simulink model "joystick_and_autonomous_control"  (Simulink 8.2)
settings: Solver=FixedStepDiscrete  StartTime=0.0  StopTime=inf  FixedStep=0.04  RelTol=1e-3
libraries: etargetslib x17, simulink x13, dspnetwork x11, dspmtrx3 x10, xpcseriallib x7, visionsinks x2, visionstatistics x1, visiontextngfix x1, aerolibanimutils x1, SimulinkExecutionControl x1, instrumentlib x1
(part 1 of 2)
settings Model: Creator=Ballistyx  LastModifiedBy=menkh
settings DebuggingCC: MultiTaskDSMMsg=warning  MultiTaskCondExecSysMsg=none  FcnCallInpInsideContextMsg=EnableAllAsWarning
settings RTWCC: IncludeERTFirstTime=on
settings GRTTargetCC: CombineOutputUpdateFcns=on  GRTInterface=off

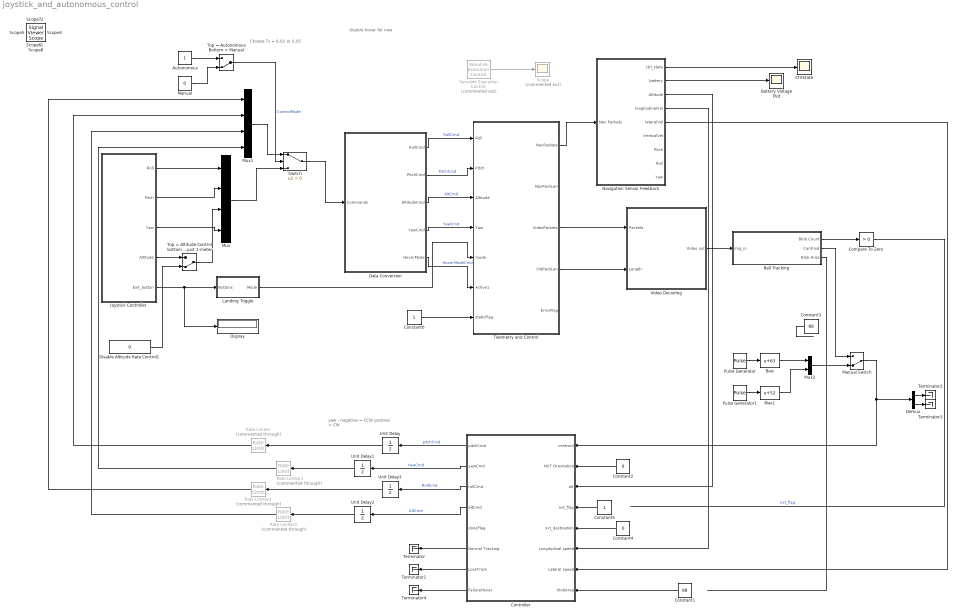
== system joystick_and_autonomous_control ==
  note: Choose Ts = 0.02 or 0.05
  note: yaw - negative = CCW
      | positive = CW
  note: disable hover for now
  Autonomous : Constant
  Ball Tracking : Subsystem
  Battery Voltage Plot : Scope
  Bias : Bias  Bias=63
  Bias1 : Bias  Bias=52  SaturateOnIntegerOverflow=on
  Compare To Zero : simulink/Logic and Bit Operations/Compare To Zero  relop=>  OutDataTypeStr=boolean
  Constant1 : Constant  Value=88
  Constant2 : Constant  Value=0
  Constant3 : Constant  Value=88
  Constant4 : Constant  Value=0  OutDataTypeStr=boolean
  Constant5 : Constant  OutDataTypeStr=boolean
  Constant6 : Constant  OutDataTypeStr=boolean
  "Controller " : Subsystem
  CtrlState : Scope
      settings: YMin=124518  YMax=137626  SaveName=ScopeData2
  Data Conversion : Subsystem
  Demux : Demux  Outputs=2
  Disable Altitude Rate Control1 : Constant  Value=0
  Display : Display
  Joystick Controller : Subsystem
  Landing Toggle : Subsystem
  Manual : Constant  Value=0
  Manual Switch : ManualSwitch  CurrentSetting=0
  Mux : Mux
  Mux1 : Mux
  Mux2 : Mux  Inputs=2
  Navigation Sensor Feedback : Subsystem
  Pulse Generator : DiscretePulseGenerator  PulseType=Time based  Amplitude=50  Period=6  PulseWidth=50
  Pulse Generator1 : DiscretePulseGenerator  PulseType=Time based  Amplitude=40  Period=6  PulseWidth=50  PhaseDelay=3
  Rate Limiter{,1..3} (4 alike) : RateLimiter  Commented=through  RisingSlewLimit=0.2  FallingSlewLimit=-0.2  SampleTimeMode=inherited
  Scope : Scope  Commented=on
  Simulink Execution Control : SimulinkExecutionControl/Simulink Execution Control  Commented=on  proc_pri=NORMAL_PRIORITY_CLASS  thread_pri=THREAD_PRIORITY_NORMAL  rt_sim=on  factor=1  ovrrun=Continue execution  Ts=-1
  Switch : Switch  Criteria=u2 > Threshold
  Telemetry and Control : Stateflow chart  TreatAsAtomicUnit=on
  Terminator{,1..4} (5 alike) : Terminator
  Top = Altitude Control bottom = Auto adjust 1-meter : ManualSwitch  CurrentSetting=0
  Top = Autonomous Bottom = Manual : ManualSwitch  CurrentSetting=0
  Unit Delay{,1..3} (4 alike) : UnitDelay  SampleTime=-1
  Video Decoding : Subsystem
  Scope1 : SignalViewerScope  IOType=viewer  NumInputPorts=2  RefreshTime=0.035000
      settings: YMin=-5~-5  YMax=5~5
  Scope2 : SignalViewerScope  IOType=viewer  NumInputPorts=5  ZoomMode=xonly  LegendLocations=|  RefreshTime=0.035000
      | 0.70961     0.93174     0.26029    0.024351
      | 0.70961     0.74251     0.26029    0.024351
      | 0.83444     0.55449     0.13546    0.024351
      | 0.83444     0.36647     0.13546    0.024351
      | 0.83444     0.15848     0.13546    0.043114
      settings: ShowLegends=on  TimeRange=60  YMin=0~0~-1~-1~-250  YMax=60~2~2~2~2750
  Scope3 : SignalViewerScope  IOType=viewer  NumInputPorts=6  ZoomMode=yonly  RefreshTime=0.035000
      settings: TimeRange=10  YMin=84.55~69.34999999999999~-1.05~-1~-1~-1  YMax=93.45~76.65000000000001~-0.95~1~1~1  SaveName=ScopeData2
  Scope4 : SignalViewerScope  IOType=viewer  NumInputPorts=6  ZoomMode=xonly  RefreshTime=0.035000
      settings: TimeRange=30.38297872340426  YMin=-0.2~-1~-0.2~0~0~0  YMax=0.2~1~0.2~0.06~150~150  SaveName=ScopeData3
  Scope5 : SignalViewerScope  IOType=viewer  NumInputPorts=3  ZoomMode=xonly  RefreshTime=0.035000
      settings: YMin=-1~-1~-1  YMax=1~1~1  SaveName=ScopeData4
  Scope6 : SignalViewerScope  IOType=viewer  NumInputPorts=6  ZoomMode=xonly  RefreshTime=0.035000
      settings: YMin=-5~-5~-5~-5~-5~-5  YMax=5~5~5~5~5~5  SaveName=ScopeData5
  Scope7 : SignalViewerScope  IOType=viewer  NumInputPorts=4  RefreshTime=0.035000
      settings: YMin=-5~-5~-5~-5  YMax=5~5~5~5  SaveName=ScopeData6
  Scope8 : SignalViewerScope  IOType=viewer  RefreshTime=0.035000
      settings: TimeRange=30  YMin=-2  YMax=2  SaveName=ScopeData7
  wires:
  Data Conversion/5(HoverMode) -> Telemetry and Control/6(Active1)  "HoverModeCmd"
  Telemetry and Control/4(VidPackLen) -> Video Decoding/2(Length)
  Data Conversion/2(PitchCmd) -> Telemetry and Control/2(Pitch)  "PitchCmd"
  Data Conversion/1(RollCmd) -> Telemetry and Control/1(Roll)  "RollCmd"
  Telemetry and Control/3(VideoPackets) -> Video Decoding/1(Packets)
  Simulink Execution Control/1 -> Scope/1
  Landing Toggle/1(Mode) -> Telemetry and Control/5(mode)
  Telemetry and Control/1(NavPackets) -> Navigation Sensor Feedback/1(Nav Packets)
  Data Conversion/4(YawCmd) -> Telemetry and Control/4(Yaw)  "YawCmd"
  Data Conversion/3(AltitudeCmd) -> Telemetry and Control/3(Altitude)  "AltCmd"
  Joystick Controller/5(Exit_button) -> Display/1, Landing Toggle/1(Buttons)
  Joystick Controller/1(Roll) -> Mux/1
  Joystick Controller/2(Pitch) -> Mux/2
  Joystick Controller/3(Yaw) -> Mux/4
  Mux1/1 -> Switch/1
  Navigation Sensor Feedback/3(Altitude) -> "Controller "/3(alt)
  Joystick Controller/4(Altitude) -> Top = Altitude Control bottom = Auto adjust 1-meter/1
  Top = Altitude Control bottom = Auto adjust 1-meter/1 -> Mux/3
  Disable Altitude Rate Control1/1 -> Top = Altitude Control bottom = Auto adjust 1-meter/2
  "Controller "/1(pitchCmd) -> Unit Delay/1  "pitchCmd"
  "Controller "/2(yawCmd) -> Unit Delay1/1  "YawCmd"
  "Controller "/3(rollCmd) -> Unit Delay3/1  "RollCmd"
  "Controller "/4(altCmd) -> Unit Delay2/1  "AltCmd"
  Unit Delay/1 -> Rate Limiter/1
  Unit Delay1/1 -> Rate Limiter1/1
  Unit Delay3/1 -> Rate Limiter2/1
  Unit Delay2/1 -> Rate Limiter3/1
  Video Decoding/1(Video out) -> Ball Tracking/1(img_in)
  Constant2/1 -> "Controller "/2(NXT Orientation)
  Compare To Zero/1 -> ?  "nxt_flag"
  Constant4/1 -> "Controller "/5(nxt_destination)
  Navigation Sensor Feedback/2(battery) -> Battery Voltage Plot/1
  Navigation Sensor Feedback/1(ctrl_state) -> CtrlState/1
  Pulse Generator/1 -> Bias/1
  Bias/1 -> Mux2/1
  Pulse Generator1/1 -> Bias1/1
  Bias1/1 -> Mux2/2
  "Controller "/6(Normal Tracking) -> Terminator/1
  Mux2/1 -> Manual Switch/2
  Ball Tracking/2(Centroid) -> Manual Switch/1
  Constant3/1 -> ?
  "Controller "/7(LossTrack) -> Terminator1/1
  Manual Switch/1 -> Demux/1, "Controller "/1(centroid)
  Demux/1 -> Terminator2/1
  Demux/2 -> Terminator3/1
  Navigation Sensor Feedback/4(longitudinalVel) -> "Controller "/6(Longitudinal speed)
  Navigation Sensor Feedback/5(lateralVel) -> "Controller "/7(Lateral speed)
  Ball Tracking/1(Blob Count) -> Compare To Zero/1
  Rate Limiter/1 -> Mux1/2
  Rate Limiter1/1 -> Mux1/4
  Rate Limiter2/1 -> Mux1/1
  Rate Limiter3/1 -> Mux1/3
  "Controller "/8(FailureHover) -> Terminator4/1
  Autonomous/1 -> Top = Autonomous Bottom = Manual/1
  Manual/1 -> Top = Autonomous Bottom = Manual/2
  Mux/1 -> Switch/3
  Switch/1 -> Data Conversion/1(Commands)
  Top = Autonomous Bottom = Manual/1 -> Switch/2  "ControlMode"
  Constant1/1 -> "Controller "/8(blobArea)
  Ball Tracking/3(Blob Area) -> ?
  Constant5/1 -> "Controller "/4(nxt_flag)
  Constant6/1 -> Telemetry and Control/7(staticFlag)

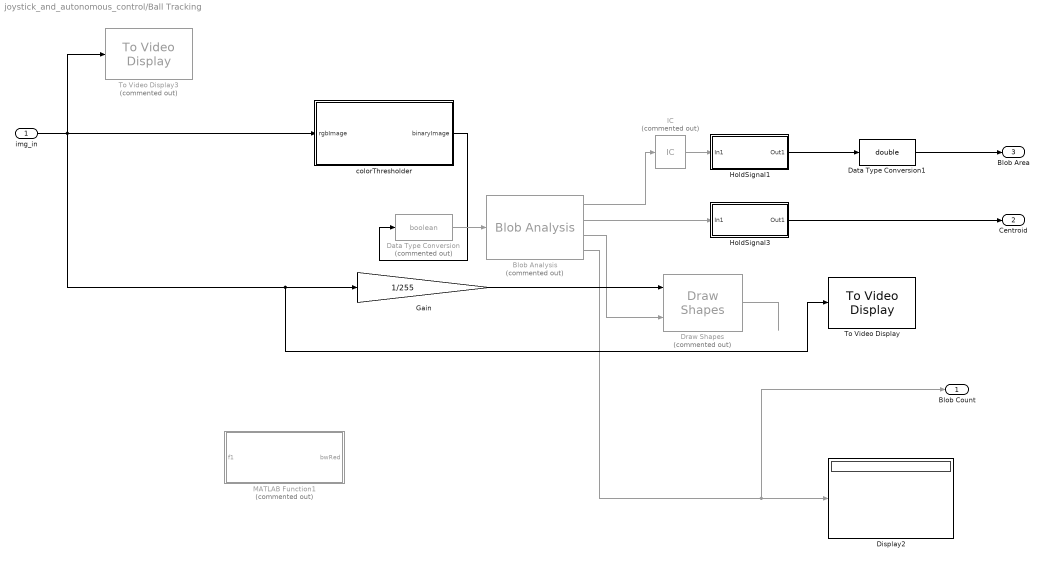
== system joystick_and_autonomous_control/Ball Tracking ==
  img_in : Inport
  Blob Analysis : visionstatistics/Blob Analysis  Tag=vipblks_row_conv  Commented=on  area=on  centroid=on  bBox=on  majorAxis=off  minorAxis=off  angle=off  eccentricity=off  equivDiameterSq=off  extent=off  perimeter=off  maxBlobs=1  warnIfNumBlobsExceeded=off  isCount=on  useMinArea=on  minArea=30  useMaxArea=off  maxArea=intmax('uint32')  excludeBorderBlob=off  outDT=double  isOutVarDim=off  isFill=on  fillValues=-1  conn=8  isLabel=off  outputMode=Binary point scaling  outputWordLength=32  outputFracLength=16  firstCoeffMode=Binary point scaling  firstCoeffWordLength=16  firstCoeffFracLength=14  secondCoeffMode=Binary point scaling  secondCoeffWordLength=32  secondCoeffFracLength=16  accumMode=Binary point scaling  accumWordLength=32  accumFracLength=0  prodOutputMode=Binary point scaling  prodOutputWordLength=32  prodOutputFracLength=16  roundingMode=Floor  overflowMode=off
  Data Type Conversion : DataTypeConversion  Commented=on  OutDataTypeStr=boolean
  Data Type Conversion1 : DataTypeConversion  OutDataTypeStr=double
  Display2 : Display
  Draw Shapes : visiontextngfix/Draw Shapes  Commented=on  shape=Rectangles  fill=off  fillClrSource=Specify via dialog  display=White  intensity=200  color=[200 255 100]  opacity=0.6  viewport=Entire image  antialiasing=off  inType=Obsolete  imagePorts=One multidimensional signal  prodOutputMode=Binary point scaling  prodOutputWordLength=32  prodOutputFracLength=14  memoryMode=Specify word length  memoryWordLength=16  memoryFracLength=15  roundingMode=Floor  overflowMode=off
  Gain : Gain  Gain=1/255
  HoldSignal1 : Subsystem
  HoldSignal3 : Subsystem
  IC : InitialCondition  Commented=on  Value=600
  MATLAB Function1 : MATLAB Function  Commented=on  TreatAsAtomicUnit=on
  To Video Display : visionsinks/To Video Display  inputType=Obsolete  imagePorts=One multidimensional signal  OutputDevice=On-screen video monitor  fullScreen=off  videoWindowX=64  videoWindowY=89  saveWindowSize=off  videoWindowWidth=640  videoWindowHeight=360  dataOrg=Column-major  openAtMdlStart=on  isWindowOpen=on  inputColorFormat=RGB
  To Video Display3 : visionsinks/To Video Display  Commented=on  inputType=Obsolete  imagePorts=One multidimensional signal  OutputDevice=On-screen video monitor  fullScreen=off  videoWindowX=93  videoWindowY=450  saveWindowSize=off  videoWindowWidth=176  videoWindowHeight=144  dataOrg=Column-major  openAtMdlStart=on  isWindowOpen=off  inputColorFormat=RGB
  colorThresholder : Subsystem
  Blob Count : Outport
  Centroid : Outport  Port=2
  Blob Area : Outport  Port=3
  wires:
  Blob Analysis/3 -> Draw Shapes/2
  Draw Shapes/1 -> ?
  Blob Analysis/2 -> HoldSignal3/1(In1)
  Blob Analysis/4 -> Display2/1, Blob Count/1
  colorThresholder/1(binaryImage) -> Data Type Conversion/1
  img_in/1 -> To Video Display3/1, colorThresholder/1(rgbImage), To Video Display/1, Gain/1
  Data Type Conversion/1 -> Blob Analysis/1
  HoldSignal3/1(Out1) -> Centroid/1
  Blob Analysis/1 -> IC/1
  HoldSignal1/1(Out1) -> Data Type Conversion1/1
  Data Type Conversion1/1 -> Blob Area/1
  IC/1 -> HoldSignal1/1(In1)
  Gain/1 -> Draw Shapes/1

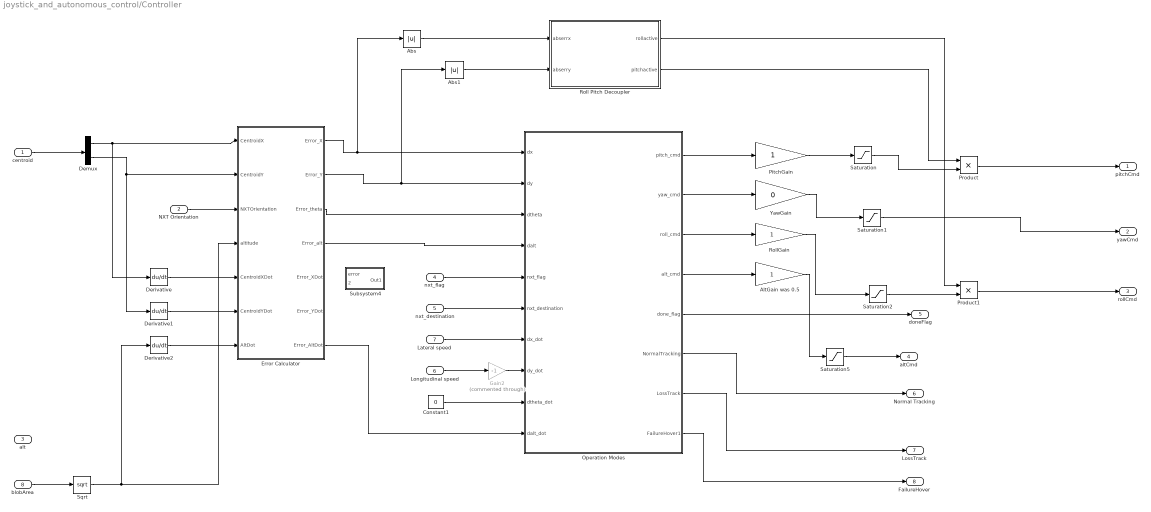
== system joystick_and_autonomous_control/Controller  ==
  centroid : Inport
  NXT Orientation : Inport  Port=2
  alt : Inport  Port=3
  nxt_flag : Inport  Port=4  OutDataTypeStr=boolean
  nxt_destination : Inport  Port=5  OutDataTypeStr=boolean
  Longitudinal speed : Inport  Port=6
  Lateral speed : Inport  Port=7
  blobArea : Inport  Port=8
  Abs : Abs
  Abs1 : Abs
  AltGain was 0.5 : Gain
  Constant1 : Constant  Value=0
  Demux : Demux  Outputs=2
  Derivative : Derivative
  Derivative1 : Derivative
  Derivative2 : Derivative
  Error Calculator : Subsystem
  Gain2 : Gain  Commented=through  Gain=-1
  Operation Modes : Stateflow chart  TreatAsAtomicUnit=on
  PitchGain : Gain
  Product : Product
  Product1 : Product
  Roll Pitch Decoupler : Stateflow chart  TreatAsAtomicUnit=on
  RollGain : Gain
  Saturation{,1..2,5} (4 alike) : Saturate  UpperLimit=1  LowerLimit=-1
  Sqrt : Sqrt  SaturateOnIntegerOverflow=on
  Subsystem4 : Subsystem
  YawGain : Gain  Gain=0
  pitchCmd : Outport
  yawCmd : Outport  Port=2
  rollCmd : Outport  Port=3
  altCmd : Outport  Port=4
  doneFlag : Outport  Port=5
  Normal Tracking : Outport  Port=6
  LossTrack : Outport  Port=7
  FailureHover : Outport  Port=8
  wires:
  Error Calculator/4(Error_alt) -> Operation Modes/4(dalt)
  Demux/2 -> Error Calculator/2(CentroidY), Derivative1/1
  Demux/1 -> Derivative/1, Error Calculator/1(CentroidX)
  centroid/1 -> Demux/1
  Saturation1/1 -> yawCmd/1
  RollGain/1 -> Saturation2/1
  Operation Modes/1(pitch_cmd) -> PitchGain/1
  Saturation2/1 -> Product1/2
  YawGain/1 -> Saturation1/1
  PitchGain/1 -> Saturation/1
  Operation Modes/3(roll_cmd) -> RollGain/1
  Saturation/1 -> Product/2
  Operation Modes/2(yaw_cmd) -> YawGain/1
  Constant1/1 -> Operation Modes/9(dtheta_dot)
  Error Calculator/3(Error_theta) -> Operation Modes/3(dtheta)
  NXT Orientation/1 -> Error Calculator/3(NXTOrientation)
  nxt_flag/1 -> Operation Modes/5(nxt_flag)
  nxt_destination/1 -> Operation Modes/6(nxt_destination)
  Operation Modes/5(done_flag) -> doneFlag/1
  Operation Modes/4(alt_cmd) -> AltGain was 0.5/1
  AltGain was 0.5/1 -> Saturation5/1
  Operation Modes/6(" NormalTracking") -> Normal Tracking/1
  Derivative/1 -> Error Calculator/5(CentroidXDot)
  Derivative1/1 -> Error Calculator/6(CentroidYDot)
  Operation Modes/7(LossTrack) -> LossTrack/1
  Saturation5/1 -> altCmd/1
  Derivative2/1 -> Error Calculator/7(AltDot)
  Error Calculator/1(Error_X) -> Operation Modes/1(dx), Abs/1
  Error Calculator/2(Error_Y) -> Operation Modes/2(dy), Abs1/1
  Lateral speed/1 -> Operation Modes/7(dx_dot)
  Longitudinal speed/1 -> Gain2/1
  Gain2/1 -> Operation Modes/8(dy_dot)
  Error Calculator/7(Error_AltDot) -> Operation Modes/10(dalt_dot)
  blobArea/1 -> Sqrt/1
  Sqrt/1 -> Derivative2/1, Error Calculator/4(altitude)
  Operation Modes/8(FailureHover1) -> FailureHover/1
  Product/1 -> pitchCmd/1
  Product1/1 -> rollCmd/1
  Abs/1 -> Roll Pitch Decoupler/1(abserrx)
  Abs1/1 -> Roll Pitch Decoupler/2(abserry)
  Roll Pitch Decoupler/2(pitchactive) -> Product/1
  Roll Pitch Decoupler/1(rollactive) -> Product1/1

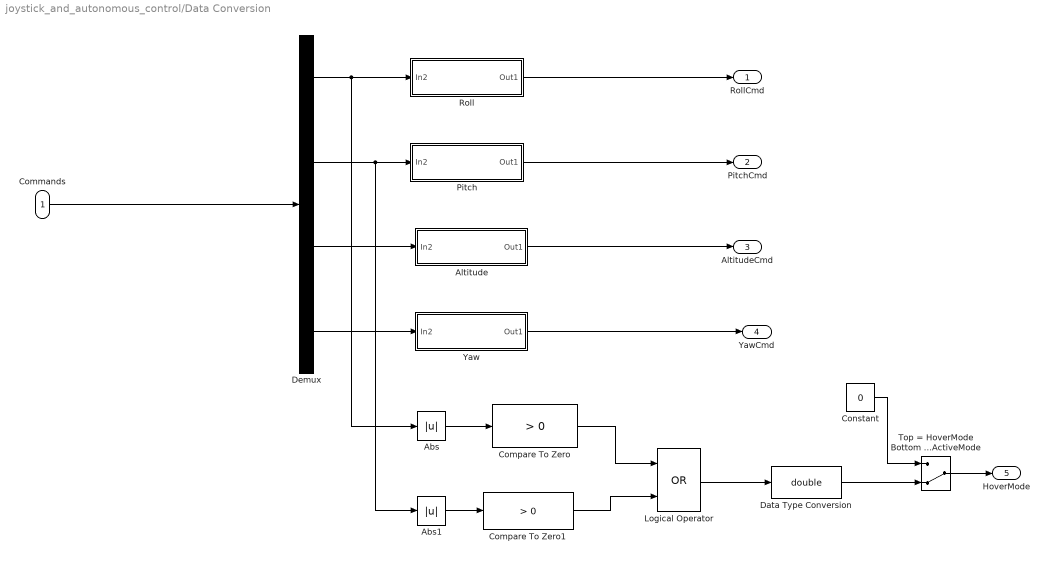
== system joystick_and_autonomous_control/Data Conversion ==
  Commands : Inport
  Abs : Abs
  Abs1 : Abs
  Altitude : Subsystem
  Compare To Zero : simulink/Logic and Bit Operations/Compare To Zero  relop=>  OutDataTypeStr=uint8
  Compare To Zero1 : simulink/Logic and Bit Operations/Compare To Zero  relop=>  OutDataTypeStr=uint8
  Constant : Constant  Value=0
  Data Type Conversion : DataTypeConversion  OutDataTypeStr=double
  Demux : Demux
  Logical Operator : Logic  Operator=OR  AllPortsSameDT=off  OutDataTypeStr=boolean
  Pitch : Subsystem
  Roll : Subsystem
  Top = HoverMode Bottom = ActiveMode : ManualSwitch  CurrentSetting=0
  Yaw : Subsystem
  RollCmd : Outport
  PitchCmd : Outport  Port=2
  AltitudeCmd : Outport  Port=3
  YawCmd : Outport  Port=4
  HoverMode : Outport  Port=5
  wires:
  Demux/1 -> Roll/1(In2), Abs/1
  Demux/2 -> Pitch/1(In2), Abs1/1
  Demux/3 -> Altitude/1(In2)
  Demux/4 -> Yaw/1(In2)
  Commands/1 -> Demux/1
  Roll/1(Out1) -> RollCmd/1
  Pitch/1(Out1) -> PitchCmd/1
  Altitude/1(Out1) -> AltitudeCmd/1
  Yaw/1(Out1) -> YawCmd/1
  Compare To Zero/1 -> Logical Operator/1
  Compare To Zero1/1 -> Logical Operator/2
  Logical Operator/1 -> Data Type Conversion/1
  Data Type Conversion/1 -> Top = HoverMode Bottom = ActiveMode/2
  Abs/1 -> Compare To Zero/1
  Abs1/1 -> Compare To Zero1/1
  Top = HoverMode Bottom = ActiveMode/1 -> HoverMode/1
  Constant/1 -> Top = HoverMode Bottom = ActiveMode/1

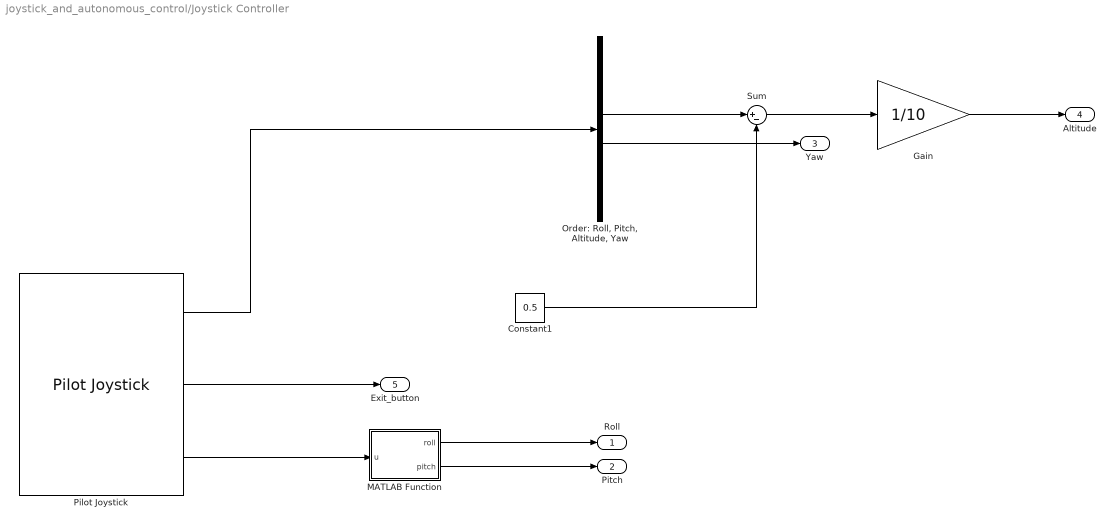
== system joystick_and_autonomous_control/Joystick Controller ==
  Constant1 : Constant  Value=0.5
  Gain : Gain  Gain=1/10
  MATLAB Function : MATLAB Function  TreatAsAtomicUnit=on
  "Order: Roll, Pitch, Altitude, Yaw" : Demux  Outputs=6
  Pilot Joystick : aerolibanimutils/Pilot Joystick  JoystickID=Joystick1  OutputConfiguration=AllOutputs  SampleTime=0.04
  Sum : Sum  Inputs=|+-
  Roll : Outport
  Pitch : Outport  Port=2
  Yaw : Outport  Port=3
  Altitude : Outport  Port=4
  Exit_button : Outport  Port=5
  wires:
  Pilot Joystick/1 -> "Order: Roll, Pitch, Altitude, Yaw"/1
  Pilot Joystick/3 -> MATLAB Function/1(u)
  "Order: Roll, Pitch, Altitude, Yaw"/3 -> Sum/1
  Constant1/1 -> Sum/2
  Sum/1 -> Gain/1
  MATLAB Function/1(roll) -> Roll/1
  MATLAB Function/2(pitch) -> Pitch/1
  Gain/1 -> Altitude/1
  "Order: Roll, Pitch, Altitude, Yaw"/4 -> Yaw/1
  Pilot Joystick/2 -> Exit_button/1

== system joystick_and_autonomous_control/Landing Toggle ==
  Buttons : Inport
  Data Type Conversion : DataTypeConversion
  Display4 : Display
  Display5 : Display
  MATLAB Function : MATLAB Function  TreatAsAtomicUnit=on
  Mode 0 : Constant  Value=0
  Mode 4 : Constant  Value=4
  Switch : Switch  Criteria=u2 > Threshold
  Unit Delay : UnitDelay  SampleTime=-1
  Unit Delay1 : UnitDelay  SampleTime=-1
  Mode : Outport
  wires:
  Unit Delay/1 -> MATLAB Function/2(add_last)
  MATLAB Function/2(adder) -> Display4/1, Unit Delay/1
  MATLAB Function/3(exit_u) -> Unit Delay1/1
  Unit Delay1/1 -> MATLAB Function/3(u_last)
  Data Type Conversion/1 -> MATLAB Function/1(u), Display5/1
  MATLAB Function/1(toggle) -> Switch/2
  Mode 4/1 -> Switch/1
  Mode 0/1 -> Switch/3
  Switch/1 -> Mode/1
  Buttons/1 -> Data Type Conversion/1

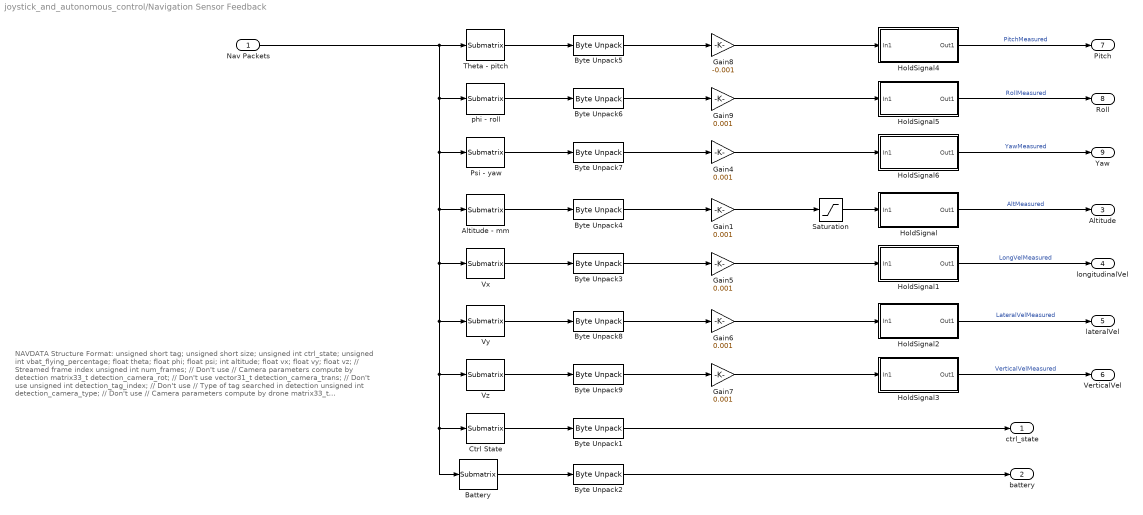
== system joystick_and_autonomous_control/Navigation Sensor Feedback ==
  note: NAVDATA Structure Format:
      |
      |         unsigned short tag;
      |         unsigned short size;
      |         unsigned int   ctrl_state;
      |         unsigned int   vbat_flying_percentage;
      |         float          theta;
      |         float          phi;
      |         float          psi;
      |         int            altitude;
      |         float          vx;
      |         float          vy;
      |         float          vz;
      |
      |         // Streamed frame index
      |         unsigned int num_frames;                // Don't use
      |
      |         // Camera parameters compute by detection
      |         matrix33_t   detection_camera_rot;      // Don't use
      |         vector31_t   detection_camera_trans;    // Don't use
      |         unsigned int detection_tag_index;       // Don't use
      |
      |         // Type of tag searched in detection
      |         unsigned int detection_camera_type;     // Don't use
      |
      |         // Camera parameters compute by drone
      |         matrix33_t drone_camera_rot;            // Don't use
      |         vector31_t drone_camera_trans;          // Don't use
  Nav Packets : Inport
  Altitude - mm : dspmtrx3/Submatrix  RowSpan=Range of rows  RowStartMode=Index  RowStartIndex=41  RowEndMode=Index  RowEndIndex=44  ColSpan=All columns  ColStartMode=Index  ColStartIndex=4  ColEndMode=Index  ColEndIndex=4
  Battery : dspmtrx3/Submatrix  RowSpan=Range of rows  RowStartMode=Index  RowStartIndex=25  RowEndMode=Index  RowEndIndex=28  ColSpan=All columns  ColStartMode=Index  ColStartIndex=4  ColEndMode=Index  ColEndIndex=4
  Byte Unpack1 : etargetslib/Byte Unpack  dimensions={[1]}  datatypes={'uint32'}  byteAlign=1
  Byte Unpack2 : etargetslib/Byte Unpack  dimensions={[1]}  datatypes={'uint32'}  byteAlign=1
  Byte Unpack{3,5..9} (6 alike) : etargetslib/Byte Unpack  dimensions={[1]}  datatypes={'single'}  byteAlign=1
  Byte Unpack4 : etargetslib/Byte Unpack  dimensions={[1]}  datatypes={'uint32'}  byteAlign=1
  Ctrl State : dspmtrx3/Submatrix  RowSpan=Range of rows  RowStartMode=Index  RowStartIndex=21  RowEndMode=Index  RowEndIndex=24  ColSpan=All columns  ColStartMode=Index  ColStartIndex=4  ColEndMode=Index  ColEndIndex=4
  Gain{1,5..7} (4 alike) : Gain  Gain=0.001  OutDataTypeStr=double
  Gain4 : Gain  Gain=0.001
  Gain8 : Gain  Gain=-0.001
  Gain9 : Gain  Gain=0.001
  HoldSignal : Subsystem
  HoldSignal1 : Subsystem
  HoldSignal2 : Subsystem
  HoldSignal3 : Subsystem
  HoldSignal4 : Subsystem
  HoldSignal5 : Subsystem
  HoldSignal6 : Subsystem
  Psi - yaw : dspmtrx3/Submatrix  RowSpan=Range of rows  RowStartMode=Index  RowStartIndex=37  RowEndMode=Index  RowEndIndex=40  ColSpan=All columns  ColStartMode=Index  ColStartIndex=4  ColEndMode=Index  ColEndIndex=4
  Saturation : Saturate  UpperLimit=10  LowerLimit=0  OutDataTypeStr=Inherit: Inherit via back propagation
  Theta - pitch : dspmtrx3/Submatrix  RowSpan=Range of rows  RowStartMode=Index  RowStartIndex=29  RowEndMode=Index  RowEndIndex=32  ColSpan=All columns  ColStartMode=Index  ColStartIndex=4  ColEndMode=Index  ColEndIndex=4
  Vx : dspmtrx3/Submatrix  RowSpan=Range of rows  RowStartMode=Index  RowStartIndex=45  RowEndMode=Index  RowEndIndex=48  ColSpan=All columns  ColStartMode=Index  ColStartIndex=4  ColEndMode=Index  ColEndIndex=4
  Vy : dspmtrx3/Submatrix  RowSpan=Range of rows  RowStartMode=Index  RowStartIndex=49  RowEndMode=Index  RowEndIndex=52  ColSpan=All columns  ColStartMode=Index  ColStartIndex=4  ColEndMode=Index  ColEndIndex=4
  Vz : dspmtrx3/Submatrix  RowSpan=Range of rows  RowStartMode=Index  RowStartIndex=53  RowEndMode=Index  RowEndIndex=56  ColSpan=All columns  ColStartMode=Index  ColStartIndex=4  ColEndMode=Index  ColEndIndex=4
  phi - roll : dspmtrx3/Submatrix  RowSpan=Range of rows  RowStartMode=Index  RowStartIndex=33  RowEndMode=Index  RowEndIndex=36  ColSpan=All columns  ColStartMode=Index  ColStartIndex=4  ColEndMode=Index  ColEndIndex=4
  ctrl_state : Outport
  battery : Outport  Port=2
  Altitude : Outport  Port=3
  longitudinalVel : Outport  Port=4
  lateralVel : Outport  Port=5
  VerticalVel : Outport  Port=6
  Pitch : Outport  Port=7
  Roll : Outport  Port=8
  Yaw : Outport  Port=9
  wires:
  Altitude - mm/1 -> Byte Unpack4/1
  Theta - pitch/1 -> Byte Unpack5/1
  phi - roll/1 -> Byte Unpack6/1
  Psi - yaw/1 -> Byte Unpack7/1
  Byte Unpack5/1 -> Gain8/1
  Byte Unpack6/1 -> Gain9/1
  Byte Unpack7/1 -> Gain4/1
  Byte Unpack4/1 -> Gain1/1
  HoldSignal4/1(Out1) -> Pitch/1  "PitchMeasured"
  HoldSignal5/1(Out1) -> Roll/1  "RollMeasured"
  Nav Packets/1 -> Psi - yaw/1, Altitude - mm/1, Vx/1, Ctrl State/1, Battery/1, Vz/1, Vy/1, phi - roll/1, Theta - pitch/1
  Ctrl State/1 -> Byte Unpack1/1
  Byte Unpack1/1 -> ctrl_state/1
  Battery/1 -> Byte Unpack2/1
  Byte Unpack2/1 -> battery/1
  Vz/1 -> Byte Unpack9/1
  Vy/1 -> Byte Unpack8/1
  Vx/1 -> Byte Unpack3/1
  Byte Unpack9/1 -> Gain7/1
  Byte Unpack8/1 -> Gain6/1
  Byte Unpack3/1 -> Gain5/1
  Gain5/1 -> HoldSignal1/1(In1)
  Gain6/1 -> HoldSignal2/1(In1)
  Gain7/1 -> HoldSignal3/1(In1)
  HoldSignal/1(Out1) -> Altitude/1  "AltMeasured"
  Saturation/1 -> HoldSignal/1(In1)
  HoldSignal3/1(Out1) -> VerticalVel/1  "VerticalVelMeasured"
  HoldSignal2/1(Out1) -> lateralVel/1  "LateralVelMeasured"
  HoldSignal1/1(Out1) -> longitudinalVel/1  "LongVelMeasured"
  Gain1/1 -> Saturation/1
  Gain8/1 -> HoldSignal4/1(In1)
  Gain9/1 -> HoldSignal5/1(In1)
  HoldSignal6/1(Out1) -> Yaw/1  "YawMeasured"
  Gain4/1 -> HoldSignal6/1(In1)

== system joystick_and_autonomous_control/Telemetry and Control/SetVideo ==
  DataStamp : Inport
  f : TriggerPort  TriggerType=function-call
      settings: CopyFcn=Stateflow.SLINSF.SimulinkMan.removeBlockPreDeleteFcn  PreDeleteFcn=Stateflow.SLINSF.SimulinkMan.unsafePredeleteFcn
  ASCII Encode 1 : xpcseriallib/ASCII Encode   format="AT*CONFIG=%d,\\\"video:video_channel\\\",\\\"0\\\"\\r"  nvars=1  maxlength=44  vartypes={ 'uint32' }
  UDP Send : dspnetwork/UDP Send  remoteURL='192.168.1.1'  remotePort=5556  localURL='0.0.0.0'  localPortSource=Specify via dialog  localPort=5556  sampletime=-1  separateLengthPort=0
  wires:
  DataStamp/1 -> ASCII Encode 1/1
  ASCII Encode 1/1 -> UDP Send/1

== system joystick_and_autonomous_control/Telemetry and Control/StartNavDemo ==
  note: Enable navdatademo
  DataStamp : Inport
  f : TriggerPort  TriggerType=function-call
      settings: CopyFcn=Stateflow.SLINSF.SimulinkMan.removeBlockPreDeleteFcn  PreDeleteFcn=Stateflow.SLINSF.SimulinkMan.unsafePredeleteFcn
  ASCII Encode 2 : xpcseriallib/ASCII Encode   format="AT*CONFIG=%d,\\\"general:navdata_demo\\\",\\\"TRUE\\\"\\r"  nvars=1  maxlength=43  vartypes={ 'uint32' }
  UDP Send1 : dspnetwork/UDP Send  remoteURL='192.168.1.1'  remotePort=5556  localURL='0.0.0.0'  localPortSource=Specify via dialog  localPort=5556  sampletime=-1  separateLengthPort=0
  wires:
  DataStamp/1 -> ASCII Encode 2/1
  ASCII Encode 2/1 -> UDP Send1/1

== system joystick_and_autonomous_control/Telemetry and Control/WakeUpNav ==
  note: set video codec
  note: wakeup nav demo
  DataStamp : Inport
  f : TriggerPort  TriggerType=function-call
      settings: CopyFcn=Stateflow.SLINSF.SimulinkMan.removeBlockPreDeleteFcn  PreDeleteFcn=Stateflow.SLINSF.SimulinkMan.unsafePredeleteFcn
  ASCII Encode 1 : xpcseriallib/ASCII Encode   format="AT*CONFIG=%d,\\\"video:video_codec\\\",\\\"32\\\"\\r"  nvars=1  maxlength=44  vartypes={ 'uint32' }
  Constant1 : Constant  OutDataTypeStr=uint8  SampleTime=-1
  UDP Send : dspnetwork/UDP Send  remoteURL='192.168.1.1'  remotePort=5556  localURL='0.0.0.0'  localPortSource=Specify via dialog  localPort=5556  sampletime=-1  separateLengthPort=0
  UDP Send1 : dspnetwork/UDP Send  remoteURL='192.168.1.1'  remotePort=5554  localURL='0.0.0.0'  localPortSource=Specify via dialog  localPort=5554  sampletime=-1  separateLengthPort=0
  wires:
  DataStamp/1 -> ASCII Encode 1/1
  Constant1/1 -> UDP Send1/1
  ASCII Encode 1/1 -> UDP Send/1

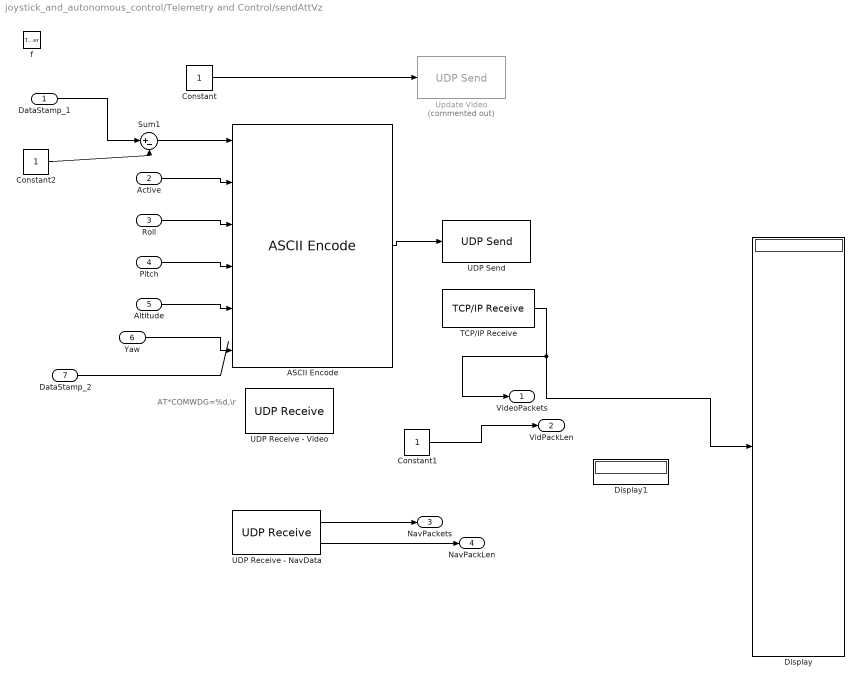
== system joystick_and_autonomous_control/Telemetry and Control/sendAttVz ==
  note: AT*COMWDG=%d,\r
  DataStamp_1 : Inport
  Active : Inport  Port=2
  Roll : Inport  Port=3
  Pitch : Inport  Port=4
  Altitude : Inport  Port=5
  Yaw : Inport  Port=6
  DataStamp_2 : Inport  Port=7
  f : TriggerPort  TriggerType=function-call
      settings: CopyFcn=Stateflow.SLINSF.SimulinkMan.removeBlockPreDeleteFcn  PreDeleteFcn=Stateflow.SLINSF.SimulinkMan.unsafePredeleteFcn
  "ASCII Encode " : xpcseriallib/ASCII Encode   format=AT*PCMD=%d,%d,%d,%d,%d,%d\r  nvars=6  maxlength=128  vartypes={ 'double' }
  Constant : Constant  Priority=12  OutDataTypeStr=uint8  SampleTime=-1
  Constant1 : Constant  Priority=12  OutDataTypeStr=uint8  SampleTime=-1
  Constant2 : Constant
  Display : Display
  Display1 : Display
  Sum1 : Sum  Inputs=|+-
  TCP/IP Receive : instrumentlib/TCP//IP Receive  Host=192.168.1.1  Port=5555  DataSize="[40000      1]"  EnableBlockingMode=on  Timeout=10  SampleTime=0.04  DataType=uint8  ByteOrder=BigEndian
  UDP Receive - NavData : dspnetwork/UDP Receive  Priority=15  localURL='0.0.0.0'  localPort=5554  remoteURL='192.168.1.1'  remotePort=-1  recvBufferSize=500  dims=500  signalDatatype=uint8  isVarSize=off  showBlockingTime=off  blockingTime=0  sampletime=-1
  UDP Receive - Video : dspnetwork/UDP Receive  Priority=16  localURL='0.0.0.0'  localPort=5555  remoteURL='192.168.1.1'  remotePort=-1  recvBufferSize=40000*2  dims=40000  signalDatatype=uint8  isVarSize=off  showBlockingTime=off  blockingTime=0  sampletime=-1
  UDP Send : dspnetwork/UDP Send  Priority=11  remoteURL='192.168.1.1'  remotePort=5556  localURL='0.0.0.0'  localPortSource=Specify via dialog  localPort=5556  sampletime=-1  separateLengthPort=0
  Update Video : dspnetwork/UDP Send  Priority=10  Commented=on  remoteURL='192.168.1.1'  remotePort=5555  localURL='0.0.0.0'  localPortSource=Specify via dialog  localPort=5555  sampletime=-1  separateLengthPort=0
  VideoPackets : Outport
  VidPackLen : Outport  Port=2  OutDataTypeStr=uint16
  NavPackets : Outport  Port=3
  NavPackLen : Outport  Port=4
  wires:
  Active/1 -> "ASCII Encode "/2
  Roll/1 -> "ASCII Encode "/3
  Pitch/1 -> "ASCII Encode "/4
  Altitude/1 -> "ASCII Encode "/5
  Yaw/1 -> "ASCII Encode "/6
  DataStamp_2/1 -> ?
  DataStamp_1/1 -> Sum1/1
  Sum1/1 -> "ASCII Encode "/1
  Constant2/1 -> Sum1/2
  "ASCII Encode "/1 -> UDP Send/1
  Constant/1 -> Update Video/1
  UDP Receive - NavData/2 -> NavPackLen/1
  TCP/IP Receive/1 -> Display/1, VideoPackets/1
  UDP Receive - NavData/1 -> NavPackets/1
  Constant1/1 -> VidPackLen/1

== system joystick_and_autonomous_control/Telemetry and Control/sendLand ==
  In1 : Inport
  f : TriggerPort  TriggerType=function-call
      settings: CopyFcn=Stateflow.SLINSF.SimulinkMan.removeBlockPreDeleteFcn  PreDeleteFcn=Stateflow.SLINSF.SimulinkMan.unsafePredeleteFcn
  "ASCII Encode " : xpcseriallib/ASCII Encode   format=AT*REF=%d,290717696\r  nvars=1  maxlength=128  vartypes={ 'double' }
  UDP Send : dspnetwork/UDP Send  remoteURL='192.168.1.1'  remotePort=5556  localURL='0.0.0.0'  localPortSource=Specify via dialog  localPort=5556  sampletime=-1  separateLengthPort=0
  wires:
  "ASCII Encode "/1 -> UDP Send/1
  In1/1 -> "ASCII Encode "/1

== system joystick_and_autonomous_control/Telemetry and Control/sendTrim ==
  DataStamp : Inport
  f : TriggerPort  TriggerType=function-call
      settings: CopyFcn=Stateflow.SLINSF.SimulinkMan.removeBlockPreDeleteFcn  PreDeleteFcn=Stateflow.SLINSF.SimulinkMan.unsafePredeleteFcn
  "ASCII Encode " : xpcseriallib/ASCII Encode   format=AT*FTRIM=%d,\r  nvars=1  maxlength=128  vartypes={ 'double' }
  UDP Send : dspnetwork/UDP Send  remoteURL='192.168.1.1'  remotePort=5556  localURL='0.0.0.0'  localPortSource=Specify via dialog  localPort=5556  sampletime=-1  separateLengthPort=0
  wires:
  DataStamp/1 -> "ASCII Encode "/1
  "ASCII Encode "/1 -> UDP Send/1

== system joystick_and_autonomous_control/Telemetry and Control/startHover ==
  note: disable hover for now
  DataStamp : Inport
  f : TriggerPort  TriggerType=function-call
      settings: CopyFcn=Stateflow.SLINSF.SimulinkMan.removeBlockPreDeleteFcn  PreDeleteFcn=Stateflow.SLINSF.SimulinkMan.unsafePredeleteFcn
  "ASCII Encode " : xpcseriallib/ASCII Encode   format=AT*REF=%d,290718208\r  nvars=1  maxlength=128  vartypes={ 'double' }
  UDP Send : dspnetwork/UDP Send  remoteURL='192.168.1.1'  remotePort=5556  localURL='0.0.0.0'  localPortSource=Specify via dialog  localPort=5556  sampletime=-1  separateLengthPort=0
  wires:
  DataStamp/1 -> "ASCII Encode "/1
  "ASCII Encode "/1 -> UDP Send/1

== system joystick_and_autonomous_control/Video Decoding ==
  Packets : Inport
  Length : Inport  Port=2
  Data Type Conversion2 : DataTypeConversion  OutDataTypeStr=uint32
  Display : Display
  Display1 : Display
  Hold Image Stream : Subsystem  TreatAsAtomicUnit=on
  S-Function2 : S-Function  FunctionName=Video_Decode  EnableBusSupport=off
  Transpose1 : dspmtrx3/Transpose  Hermitian=off  overflowFlag=off
  Video out : Outport
  wires:
  Data Type Conversion2/1 -> S-Function2/2
  Transpose1/1 -> S-Function2/1
  Packets/1 -> Display/1, Hold Image Stream/1(byte_packet_in)
  Length/1 -> Display1/1, Hold Image Stream/2(length_in), Hold Image Stream/Enable
  S-Function2/1 -> Video out/1
  Hold Image Stream/1(byte_packet_out) -> Transpose1/1
  Hold Image Stream/2(length_out) -> Data Type Conversion2/1

== system joystick_and_autonomous_control/Ball Tracking/HoldSignal1 ==
  In1 : Inport
  Compare To Zero : simulink/Logic and Bit Operations/Compare To Zero  relop=>  OutDataTypeStr=boolean
  Enabled Subsystem : Subsystem  TreatAsAtomicUnit=on
  Out1 : Outport
  wires:
  In1/1 -> Compare To Zero/1, Enabled Subsystem/1(In1)
  Compare To Zero/1 -> Enabled Subsystem/Enable
  Enabled Subsystem/1(Out1) -> Out1/1

== system joystick_and_autonomous_control/Ball Tracking/HoldSignal3 ==
  In1 : Inport
  Compare To Zero : simulink/Logic and Bit Operations/Compare To Zero  relop=>=  OutDataTypeStr=boolean
  Enabled Subsystem : Subsystem  TreatAsAtomicUnit=on
  Out1 : Outport
  wires:
  In1/1 -> Compare To Zero/1, Enabled Subsystem/1(In1)
  Compare To Zero/1 -> Enabled Subsystem/Enable
  Enabled Subsystem/1(Out1) -> Out1/1

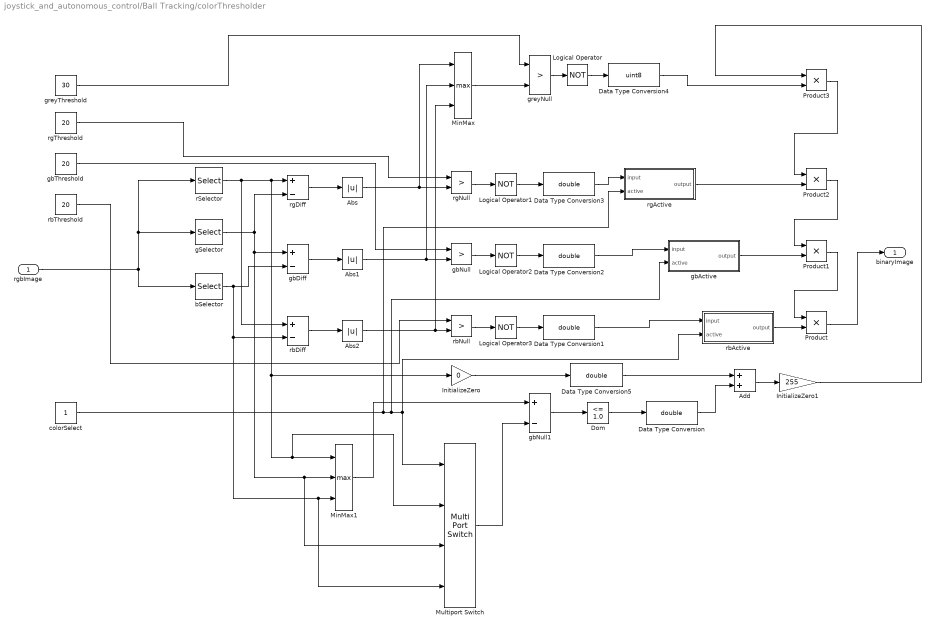
== system joystick_and_autonomous_control/Ball Tracking/colorThresholder ==
  rgbImage : Inport
  Abs : Abs
  Abs1 : Abs
  Abs2 : Abs
  Add : Sum
  Data Type Conversion{,1..3,5} (5 alike) : DataTypeConversion  OutDataTypeStr=double
  Data Type Conversion4 : DataTypeConversion  OutDataTypeStr=uint8
  Dom : simulink/Logic and Bit Operations/Compare To Constant  relop=<=  const=1.0  OutDataTypeStr=boolean
  InitializeZero : Gain  Gain=0
  InitializeZero1 : Gain  Gain=255
  Logical Operator{,1..3} (4 alike) : Logic  Operator=NOT  AllPortsSameDT=off  OutDataTypeStr=boolean
  MinMax : MinMax  Function=max  Inputs=3
  MinMax1 : MinMax  Function=max  Inputs=3
  Multiport Switch : MultiPortSwitch
  Product{,1..3} (4 alike) : Product
  bSelector : Selector  NumberOfDimensions=3  InputPortWidth=3  IndexOptions=Select all,Select all,Index vector (dialog)  Indices=[1 3],1,[3]  OutputSizes=1,1,1
  colorSelect : Constant
  gSelector : Selector  NumberOfDimensions=3  InputPortWidth=3  IndexOptions=Select all,Select all,Index vector (dialog)  Indices=[1 3],1,[2]  OutputSizes=1,1,1
  gbActive : Subsystem
  gbDiff : Sum  Inputs=+-
  gbNull : RelationalOperator  Operator=>  OutDataTypeStr=boolean
  gbNull1 : Sum  Inputs=+-
  gbThreshold : Constant  Value=20
  greyNull : RelationalOperator  Operator=>  OutDataTypeStr=boolean
  greyThreshold : Constant  Value=30
  rSelector : Selector  NumberOfDimensions=3  InputPortWidth=3  IndexOptions=Select all,Select all,Index vector (dialog)  Indices=[1 3],1,[1]  OutputSizes=1,1,1
  rbActive : Subsystem
  rbDiff : Sum  Inputs=+-
  rbNull : RelationalOperator  Operator=>  OutDataTypeStr=boolean
  rbThreshold : Constant  Value=20
  rgActive : Subsystem
  rgDiff : Sum  Inputs=+-
  "rgNull " : RelationalOperator  Operator=>  OutDataTypeStr=boolean
  rgThreshold : Constant  Value=20
  binaryImage : Outport
  wires:
  rgbImage/1 -> bSelector/1, gSelector/1, rSelector/1
  gSelector/1 -> Multiport Switch/3, MinMax1/2, gbDiff/1, rgDiff/2
  rgDiff/1 -> Abs/1
  bSelector/1 -> Multiport Switch/4, MinMax1/3, rbDiff/2, gbDiff/2
  rbDiff/1 -> Abs2/1
  gbDiff/1 -> Abs1/1
  rgThreshold/1 -> "rgNull "/1
  Abs/1 -> MinMax/1, "rgNull "/2
  gbThreshold/1 -> gbNull/1
  Abs1/1 -> MinMax/2, gbNull/2
  rbThreshold/1 -> rbNull/1
  Abs2/1 -> MinMax/3, rbNull/2
  greyThreshold/1 -> greyNull/1
  MinMax/1 -> greyNull/2
  rSelector/1 -> rbDiff/1, Multiport Switch/2, MinMax1/1, InitializeZero/1, rgDiff/1
  colorSelect/1 -> rgActive/2(active), gbActive/2(active), Multiport Switch/1, rbActive/2(active)
  MinMax1/1 -> gbNull1/1
  Multiport Switch/1 -> gbNull1/2
  gbNull1/1 -> Dom/1
  Dom/1 -> Data Type Conversion/1
  greyNull/1 -> Logical Operator/1
  "rgNull "/1 -> Logical Operator1/1
  gbNull/1 -> Logical Operator2/1
  rbNull/1 -> Logical Operator3/1
  Data Type Conversion/1 -> Add/2
  InitializeZero/1 -> Data Type Conversion5/1
  Data Type Conversion5/1 -> Add/1
  Add/1 -> InitializeZero1/1
  Logical Operator/1 -> Data Type Conversion4/1
  Logical Operator1/1 -> Data Type Conversion3/1
  Logical Operator2/1 -> Data Type Conversion2/1
  Logical Operator3/1 -> Data Type Conversion1/1
  InitializeZero1/1 -> Product3/1
  Data Type Conversion4/1 -> Product3/2
  Product3/1 -> Product2/1
  Data Type Conversion3/1 -> rgActive/1(input)
  Product2/1 -> Product1/1
  Data Type Conversion1/1 -> rbActive/1(input)
  Product/1 -> binaryImage/1
  Product1/1 -> Product/1
  Data Type Conversion2/1 -> gbActive/1(input)
  rgActive/1(output) -> Product2/2
  gbActive/1(output) -> Product1/2
  rbActive/1(output) -> Product/2

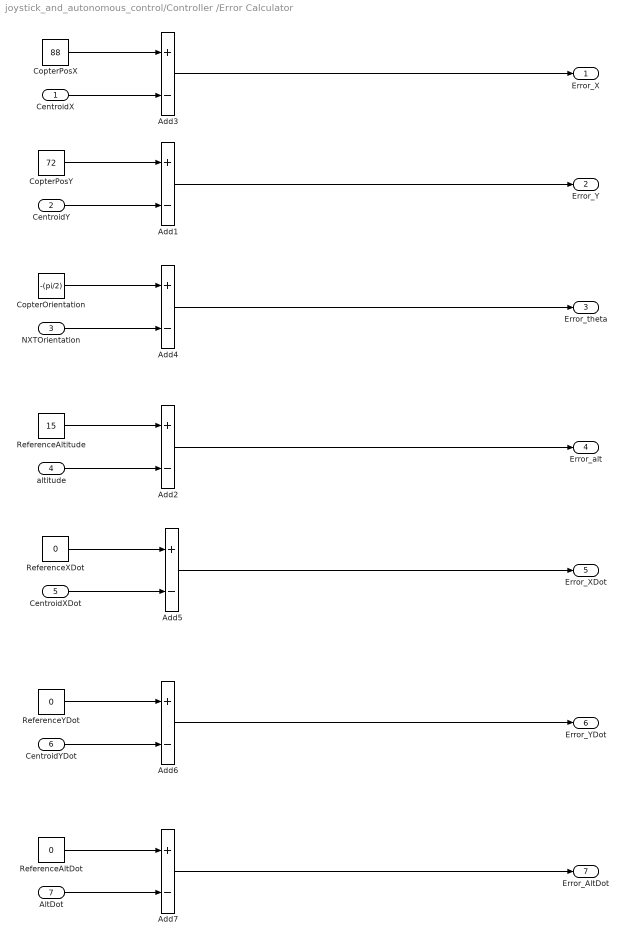
== system joystick_and_autonomous_control/Controller /Error Calculator ==
  CentroidX : Inport
  CentroidY : Inport  Port=2
  NXTOrientation : Inport  Port=3
  altitude : Inport  Port=4
  CentroidXDot : Inport  Port=5
  CentroidYDot : Inport  Port=6
  AltDot : Inport  Port=7
  Add{1..7} (7 alike) : Sum  Inputs=+-
  CopterOrientation : Constant  Value=-(pi/2)
  CopterPosX : Constant  Value=88
  CopterPosY : Constant  Value=72
  ReferenceAltDot : Constant  Value=0
  ReferenceAltitude : Constant  Value=15
  ReferenceXDot : Constant  Value=0
  ReferenceYDot : Constant  Value=0
  Error_X : Outport
  Error_Y : Outport  Port=2
  Error_theta : Outport  Port=3
  Error_alt : Outport  Port=4
  Error_XDot : Outport  Port=5
  Error_YDot : Outport  Port=6
  Error_AltDot : Outport  Port=7
  wires:
  CopterPosY/1 -> Add1/1
  CentroidY/1 -> Add1/2
  CopterPosX/1 -> Add3/1
  CentroidX/1 -> Add3/2
  Add3/1 -> Error_X/1
  Add1/1 -> Error_Y/1
  NXTOrientation/1 -> Add4/2
  CopterOrientation/1 -> Add4/1
  Add4/1 -> Error_theta/1
  ReferenceAltitude/1 -> Add2/1
  altitude/1 -> Add2/2
  Add2/1 -> Error_alt/1
  ReferenceXDot/1 -> Add5/1
  CentroidXDot/1 -> Add5/2
  Add5/1 -> Error_XDot/1
  ReferenceYDot/1 -> Add6/1
  CentroidYDot/1 -> Add6/2
  Add6/1 -> Error_YDot/1
  ReferenceAltDot/1 -> Add7/1
  AltDot/1 -> Add7/2
  Add7/1 -> Error_AltDot/1

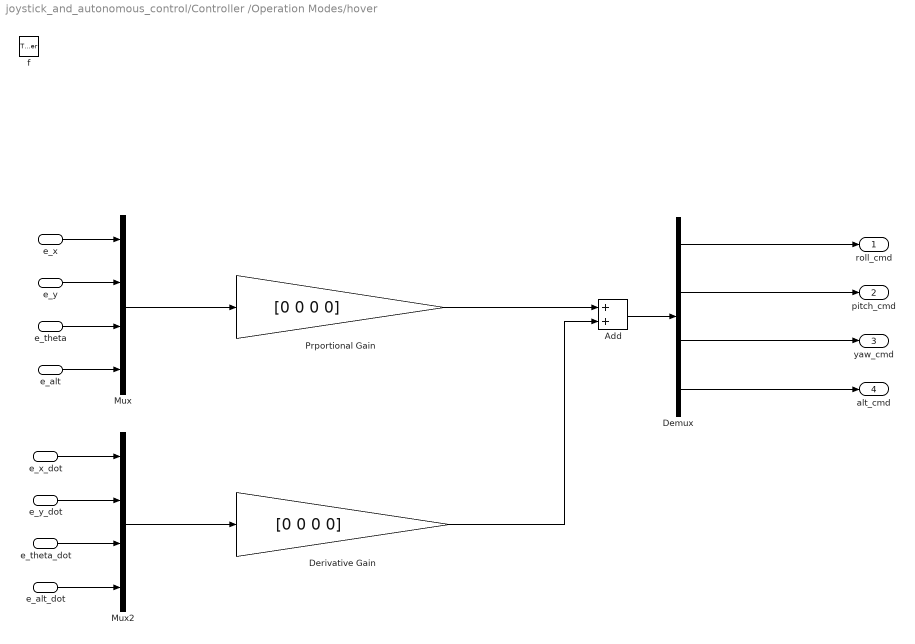
== system joystick_and_autonomous_control/Controller /Operation Modes/hover ==
  e_x : Inport
  e_y : Inport  Port=2
  e_theta : Inport  Port=3
  e_x_dot : Inport  Port=4
  e_y_dot : Inport  Port=5
  e_theta_dot : Inport  Port=6
  e_alt : Inport  Port=7
  e_alt_dot : Inport  Port=8
  f : TriggerPort  TriggerType=function-call
      settings: CopyFcn=Stateflow.SLINSF.SimulinkMan.removeBlockPreDeleteFcn  PreDeleteFcn=Stateflow.SLINSF.SimulinkMan.unsafePredeleteFcn
  Add : Sum
  Demux : Demux
  Derivative Gain : Gain  Gain=[0 0 0 0]
  Mux : Mux
  Mux2 : Mux
  Prportional Gain : Gain  Gain=[0 0 0 0]
  roll_cmd : Outport
  pitch_cmd : Outport  Port=2
  yaw_cmd : Outport  Port=3
  alt_cmd : Outport  Port=4
  wires:
  Mux/1 -> Prportional Gain/1
  e_x/1 -> Mux/1
  e_y/1 -> Mux/2
  e_theta/1 -> Mux/3
  Prportional Gain/1 -> Add/1
  Derivative Gain/1 -> Add/2
  Add/1 -> Demux/1
  Demux/3 -> yaw_cmd/1
  Demux/1 -> roll_cmd/1
  Demux/2 -> pitch_cmd/1
  Mux2/1 -> Derivative Gain/1
  e_x_dot/1 -> Mux2/1
  e_y_dot/1 -> Mux2/2
  e_theta_dot/1 -> Mux2/3
  e_alt/1 -> Mux/4
  e_alt_dot/1 -> Mux2/4
  Demux/4 -> alt_cmd/1

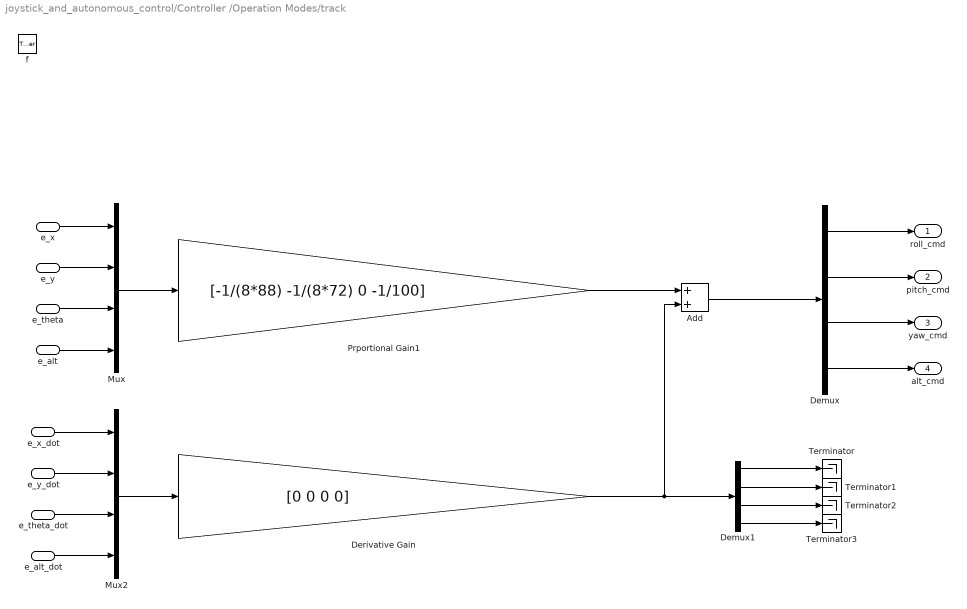
== system joystick_and_autonomous_control/Controller /Operation Modes/track ==
  e_x : Inport
  e_y : Inport  Port=2
  e_theta : Inport  Port=3
  e_x_dot : Inport  Port=4
  e_y_dot : Inport  Port=5
  e_theta_dot : Inport  Port=6
  e_alt : Inport  Port=7
  e_alt_dot : Inport  Port=8
  f : TriggerPort  TriggerType=function-call
      settings: CopyFcn=Stateflow.SLINSF.SimulinkMan.removeBlockPreDeleteFcn  PreDeleteFcn=Stateflow.SLINSF.SimulinkMan.unsafePredeleteFcn
  Add : Sum
  Demux : Demux
  Demux1 : Demux
  Derivative Gain : Gain  Gain=[0 0 0 0]
  Mux : Mux
  Mux2 : Mux
  Prportional Gain1 : Gain  Gain=[-1/(8*88) -1/(8*72) 0 -1/100]
  Terminator{,1..3} (4 alike) : Terminator
  roll_cmd : Outport
  pitch_cmd : Outport  Port=2
  yaw_cmd : Outport  Port=3
  alt_cmd : Outport  Port=4
  wires:
  e_x/1 -> Mux/1
  e_y/1 -> Mux/2
  e_theta/1 -> Mux/3
  Add/1 -> Demux/1
  Demux/3 -> yaw_cmd/1
  Demux/1 -> roll_cmd/1
  Demux/2 -> pitch_cmd/1
  Mux2/1 -> Derivative Gain/1
  e_x_dot/1 -> Mux2/1
  e_y_dot/1 -> Mux2/2
  e_theta_dot/1 -> Mux2/3
  e_alt/1 -> Mux/4
  e_alt_dot/1 -> Mux2/4
  Demux/4 -> alt_cmd/1
  Demux1/3 -> Terminator2/1
  Demux1/1 -> Terminator/1
  Demux1/2 -> Terminator1/1
  Demux1/4 -> Terminator3/1
  Mux/1 -> Prportional Gain1/1
  Prportional Gain1/1 -> Add/1
  Derivative Gain/1 -> Add/2, Demux1/1

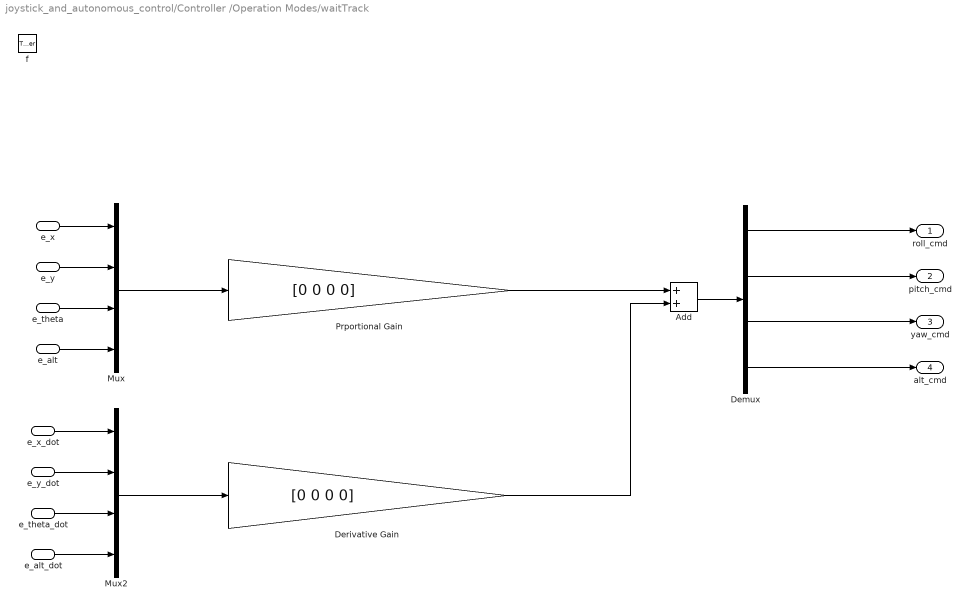
== system joystick_and_autonomous_control/Controller /Operation Modes/waitTrack ==
  e_x : Inport
  e_y : Inport  Port=2
  e_theta : Inport  Port=3
  e_x_dot : Inport  Port=4
  e_y_dot : Inport  Port=5
  e_theta_dot : Inport  Port=6
  e_alt : Inport  Port=7
  e_alt_dot : Inport  Port=8
  f : TriggerPort  TriggerType=function-call
      settings: CopyFcn=Stateflow.SLINSF.SimulinkMan.removeBlockPreDeleteFcn  PreDeleteFcn=Stateflow.SLINSF.SimulinkMan.unsafePredeleteFcn
  Add : Sum
  Demux : Demux
  Derivative Gain : Gain  Gain=[0 0 0 0]
  Mux : Mux
  Mux2 : Mux
  Prportional Gain : Gain  Gain=[0 0 0 0]
  roll_cmd : Outport
  pitch_cmd : Outport  Port=2
  yaw_cmd : Outport  Port=3
  alt_cmd : Outport  Port=4
  wires:
  Mux/1 -> Prportional Gain/1
  e_x/1 -> Mux/1
  e_y/1 -> Mux/2
  e_theta/1 -> Mux/3
  Prportional Gain/1 -> Add/1
  Derivative Gain/1 -> Add/2
  Add/1 -> Demux/1
  Demux/3 -> yaw_cmd/1
  Demux/1 -> roll_cmd/1
  Demux/2 -> pitch_cmd/1
  Mux2/1 -> Derivative Gain/1
  e_x_dot/1 -> Mux2/1
  e_y_dot/1 -> Mux2/2
  e_theta_dot/1 -> Mux2/3
  e_alt/1 -> Mux/4
  e_alt_dot/1 -> Mux2/4
  Demux/4 -> alt_cmd/1

== system joystick_and_autonomous_control/Controller /Subsystem4 ==
  error : Inport
  error_dot : Inport  Port=2
  Abs : Abs
  Constant : Constant  Value=0
  Switch : Switch  Threshold=20
  Out1 : Outport
  wires:
  error_dot/1 -> Switch/1
  error/1 -> Abs/1
  Abs/1 -> Switch/2
  Switch/1 -> Out1/1
  Constant/1 -> Switch/3

== system joystick_and_autonomous_control/Data Conversion/Altitude ==
  note: Why is this needed?
      | -According to the manual:
      |
      | Syntax:AT*PCMD_MAG=%d,%d,%d,%d,%d,%d,%d,<CR>
      | Enter a floating value between -1 and 1
      |
      | This is essentially saying: pass in a floating number (ie: single data type in MATLAB) but express it in integer form (%d).
      | the above data conversion does this and does not truncate all the bytes, this is similar to the typecast( ) function in MATLAB
  In2 : Inport
  Byte Pack : etargetslib/Byte Pack  datatypes={'single'}  byteAlign=1
  Byte Unpack : etargetslib/Byte Unpack  dimensions={[1]}  datatypes={'int32'}  byteAlign=1
  Data Type Conversion : DataTypeConversion  OutDataTypeStr=double
  Data Type Conversion2 : DataTypeConversion  OutDataTypeStr=single
  Out1 : Outport
  wires:
  Byte Pack/1 -> Byte Unpack/1
  Byte Unpack/1 -> Data Type Conversion/1
  In2/1 -> Data Type Conversion2/1
  Data Type Conversion2/1 -> Byte Pack/1
  Data Type Conversion/1 -> Out1/1

== system joystick_and_autonomous_control/Data Conversion/Pitch ==
  note: Why is this needed?
      | -According to the manual:
      |
      | Syntax:AT*PCMD_MAG=%d,%d,%d,%d,%d,%d,%d,<CR>
      | Enter a floating value between -1 and 1
      |
      | This is essentially saying: pass in a floating number (ie: single data type in MATLAB) but express it in integer form (%d).
      | the above data conversion does this and does not truncate all the bytes, this is similar to the typecast( ) function in MATLAB
  In2 : Inport
  Byte Pack : etargetslib/Byte Pack  datatypes={'single'}  byteAlign=1
  Byte Unpack : etargetslib/Byte Unpack  dimensions={[1]}  datatypes={'int32'}  byteAlign=1
  Data Type Conversion : DataTypeConversion  OutDataTypeStr=double
  Data Type Conversion2 : DataTypeConversion  OutDataTypeStr=single
  Out1 : Outport
  wires:
  Byte Pack/1 -> Byte Unpack/1
  Byte Unpack/1 -> Data Type Conversion/1
  In2/1 -> Data Type Conversion2/1
  Data Type Conversion2/1 -> Byte Pack/1
  Data Type Conversion/1 -> Out1/1

== system joystick_and_autonomous_control/Data Conversion/Roll ==
  note: Why is this needed?
      | -According to the manual:
      |
      | Syntax:AT*PCMD_MAG=%d,%d,%d,%d,%d,%d,%d,<CR>
      | Enter a floating value between -1 and 1
      |
      | This is essentially saying: pass in a floating number (ie: single data type in MATLAB) but express it in integer form (%d).
      | the above data conversion does this and does not truncate all the bytes, this is similar to the typecast( ) function in MATLAB
  In2 : Inport
  Byte Pack : etargetslib/Byte Pack  datatypes={'single'}  byteAlign=1
  Byte Unpack : etargetslib/Byte Unpack  dimensions={[1]}  datatypes={'int32'}  byteAlign=1
  Constant : Constant
  Data Type Conversion : DataTypeConversion  OutDataTypeStr=double
  Data Type Conversion2 : DataTypeConversion  OutDataTypeStr=single
  Display : Display
  Display1 : Display
  Out1 : Outport
  wires:
  In2/1 -> Data Type Conversion2/1
  Data Type Conversion2/1 -> Byte Pack/1
  Data Type Conversion/1 -> Out1/1
  Byte Pack/1 -> Byte Unpack/1, Display1/1
  Byte Unpack/1 -> Data Type Conversion/1
  ? -> Display/1

== system joystick_and_autonomous_control/Data Conversion/Yaw ==
  note: Why is this needed?
      | -According to the manual:
      |
      | Syntax:AT*PCMD_MAG=%d,%d,%d,%d,%d,%d,%d,<CR>
      | Enter a floating value between -1 and 1
      |
      | This is essentially saying: pass in a floating number (ie: single data type in MATLAB) but express it in integer form (%d).
      | the above data conversion does this and does not truncate all the bytes, this is similar to the typecast( ) function in MATLAB
  In2 : Inport
  Byte Pack : etargetslib/Byte Pack  datatypes={'single'}  byteAlign=1
  Byte Unpack : etargetslib/Byte Unpack  dimensions={[1]}  datatypes={'int32'}  byteAlign=1
  Data Type Conversion : DataTypeConversion  OutDataTypeStr=double
  Data Type Conversion2 : DataTypeConversion  OutDataTypeStr=single
  Out1 : Outport
  wires:
  Byte Pack/1 -> Byte Unpack/1
  Byte Unpack/1 -> Data Type Conversion/1
  In2/1 -> Data Type Conversion2/1
  Data Type Conversion2/1 -> Byte Pack/1
  Data Type Conversion/1 -> Out1/1

== system joystick_and_autonomous_control/Navigation Sensor Feedback/HoldSignal ==
  In1 : Inport
  Abs : Abs
  Compare To Zero : simulink/Logic and Bit Operations/Compare To Zero  relop=>  OutDataTypeStr=boolean
  Enabled Subsystem : Subsystem  TreatAsAtomicUnit=on
  Out1 : Outport
  wires:
  In1/1 -> Enabled Subsystem/1(In1), Abs/1
  Enabled Subsystem/1(Out1) -> Out1/1
  Compare To Zero/1 -> Enabled Subsystem/Enable
  Abs/1 -> Compare To Zero/1

== system joystick_and_autonomous_control/Navigation Sensor Feedback/HoldSignal1 ==
  In1 : Inport
  Abs : Abs
  Compare To Zero : simulink/Logic and Bit Operations/Compare To Zero  relop=>  OutDataTypeStr=boolean
  Enabled Subsystem : Subsystem  TreatAsAtomicUnit=on
  Out1 : Outport
  wires:
  Abs/1 -> Compare To Zero/1
  Compare To Zero/1 -> Enabled Subsystem/Enable
  Enabled Subsystem/1(Out1) -> Out1/1
  In1/1 -> Abs/1, Enabled Subsystem/1(In1)

== system joystick_and_autonomous_control/Navigation Sensor Feedback/HoldSignal2 ==
  In1 : Inport
  Abs : Abs
  Compare To Zero : simulink/Logic and Bit Operations/Compare To Zero  relop=>  OutDataTypeStr=boolean
  Enabled Subsystem : Subsystem  TreatAsAtomicUnit=on
  Out1 : Outport
  wires:
  In1/1 -> Enabled Subsystem/1(In1), Abs/1
  Enabled Subsystem/1(Out1) -> Out1/1
  Compare To Zero/1 -> Enabled Subsystem/Enable
  Abs/1 -> Compare To Zero/1

== system joystick_and_autonomous_control/Navigation Sensor Feedback/HoldSignal3 ==
  In1 : Inport
  Abs : Abs
  Compare To Zero : simulink/Logic and Bit Operations/Compare To Zero  relop=>  OutDataTypeStr=boolean
  Enabled Subsystem : Subsystem  TreatAsAtomicUnit=on
  Out1 : Outport
  wires:
  Abs/1 -> Compare To Zero/1
  Compare To Zero/1 -> Enabled Subsystem/Enable
  Enabled Subsystem/1(Out1) -> Out1/1
  In1/1 -> Abs/1, Enabled Subsystem/1(In1)

== system joystick_and_autonomous_control/Navigation Sensor Feedback/HoldSignal4 ==
  In1 : Inport
  Abs : Abs
  Compare To Zero : simulink/Logic and Bit Operations/Compare To Zero  relop=>  OutDataTypeStr=boolean
  Enabled Subsystem : Subsystem  TreatAsAtomicUnit=on
  Out1 : Outport
  wires:
  In1/1 -> Enabled Subsystem/1(In1), Abs/1
  Enabled Subsystem/1(Out1) -> Out1/1
  Compare To Zero/1 -> Enabled Subsystem/Enable
  Abs/1 -> Compare To Zero/1

== system joystick_and_autonomous_control/Navigation Sensor Feedback/HoldSignal5 ==
  In1 : Inport
  Abs : Abs
  Compare To Zero : simulink/Logic and Bit Operations/Compare To Zero  relop=>  OutDataTypeStr=boolean
  Enabled Subsystem : Subsystem  TreatAsAtomicUnit=on
  Out1 : Outport
  wires:
  In1/1 -> Enabled Subsystem/1(In1), Abs/1
  Enabled Subsystem/1(Out1) -> Out1/1
  Compare To Zero/1 -> Enabled Subsystem/Enable
  Abs/1 -> Compare To Zero/1

== system joystick_and_autonomous_control/Navigation Sensor Feedback/HoldSignal6 ==
  In1 : Inport
  Abs : Abs
  Compare To Zero : simulink/Logic and Bit Operations/Compare To Zero  relop=>  OutDataTypeStr=boolean
  Enabled Subsystem : Subsystem  TreatAsAtomicUnit=on
  Out1 : Outport
  wires:
  In1/1 -> Enabled Subsystem/1(In1), Abs/1
  Enabled Subsystem/1(Out1) -> Out1/1
  Compare To Zero/1 -> Enabled Subsystem/Enable
  Abs/1 -> Compare To Zero/1

== system joystick_and_autonomous_control/Video Decoding/Hold Image Stream ==
  byte_packet_in : Inport
  length_in : Inport  Port=2
  Enable : EnablePort
  byte_packet_out : Outport
  length_out : Outport  Port=2
  wires:
  byte_packet_in/1 -> byte_packet_out/1
  length_in/1 -> length_out/1

== system joystick_and_autonomous_control/Ball Tracking/HoldSignal1/Enabled Subsystem ==
  In1 : Inport
  Enable : EnablePort
  Out1 : Outport
  wires:
  In1/1 -> Out1/1

== system joystick_and_autonomous_control/Ball Tracking/HoldSignal3/Enabled Subsystem ==
  In1 : Inport
  Enable : EnablePort
  Out1 : Outport
  wires:
  In1/1 -> Out1/1

== system joystick_and_autonomous_control/Ball Tracking/colorThresholder/gbActive ==
  input : Inport
  active : Inport  Port=2
  Bias : Bias  Bias=1
  Constant : Constant  Value=0
  Constant1 : Constant
  Constant2 : Constant
  Gain : Gain  Gain=0  ParamDataTypeStr=uint8
  Multiport Switch : MultiPortSwitch
  Switch : Switch  Criteria=u2 ~= 0
  output : Outport
  wires:
  input/1 -> Gain/1, Switch/1
  active/1 -> Multiport Switch/1
  Switch/1 -> output/1
  Bias/1 -> Switch/3
  Gain/1 -> Bias/1
  Constant2/1 -> Multiport Switch/4
  Constant1/1 -> Multiport Switch/3
  Constant/1 -> Multiport Switch/2
  Multiport Switch/1 -> Switch/2

== system joystick_and_autonomous_control/Ball Tracking/colorThresholder/rbActive ==
  input : Inport
  active : Inport  Port=2
  Bias : Bias  Bias=1
  Constant : Constant
  Constant1 : Constant  Value=0
  Constant2 : Constant
  Gain : Gain  Gain=0
  Multiport Switch : MultiPortSwitch
  Switch : Switch  Criteria=u2 ~= 0
  output : Outport
  wires:
  input/1 -> Switch/1, Gain/1
  active/1 -> Multiport Switch/1
  Switch/1 -> output/1
  Bias/1 -> Switch/3
  Gain/1 -> Bias/1
  Constant2/1 -> Multiport Switch/4
  Constant1/1 -> Multiport Switch/3
  Constant/1 -> Multiport Switch/2
  Multiport Switch/1 -> Switch/2

== system joystick_and_autonomous_control/Ball Tracking/colorThresholder/rgActive ==
  input : Inport
  active : Inport  Port=2
  Bias : Bias  Bias=1
  Constant : Constant
  Constant1 : Constant
  Constant2 : Constant  Value=0
  Gain : Gain  Gain=0
  Multiport Switch : MultiPortSwitch
  Switch : Switch  Criteria=u2 ~= 0
  output : Outport
  wires:
  input/1 -> Gain/1, Switch/1
  active/1 -> Multiport Switch/1
  Switch/1 -> output/1
  Bias/1 -> Switch/3
  Gain/1 -> Bias/1
  Constant2/1 -> Multiport Switch/4
  Constant1/1 -> Multiport Switch/3
  Constant/1 -> Multiport Switch/2
  Multiport Switch/1 -> Switch/2

== system joystick_and_autonomous_control/Navigation Sensor Feedback/HoldSignal/Enabled Subsystem ==
  In1 : Inport
  Enable : EnablePort
  Out1 : Outport
  wires:
  In1/1 -> Out1/1

== system joystick_and_autonomous_control/Navigation Sensor Feedback/HoldSignal1/Enabled Subsystem ==
  In1 : Inport
  Enable : EnablePort
  Out1 : Outport
  wires:
  In1/1 -> Out1/1

== system joystick_and_autonomous_control/Navigation Sensor Feedback/HoldSignal2/Enabled Subsystem ==
  In1 : Inport
  Enable : EnablePort
  Out1 : Outport
  wires:
  In1/1 -> Out1/1
